simulink model "interface_model"  (R2017b)
settings: Solver=FixedStepDiscrete  StartTime=0.0  StopTime=inf  RelTol=1e-3
undefined symbols (not defined in the file or in its folder): ip
libraries: zynqradiolib x2
settings Model: Creator=tcollins  LastModifiedBy=tcollins

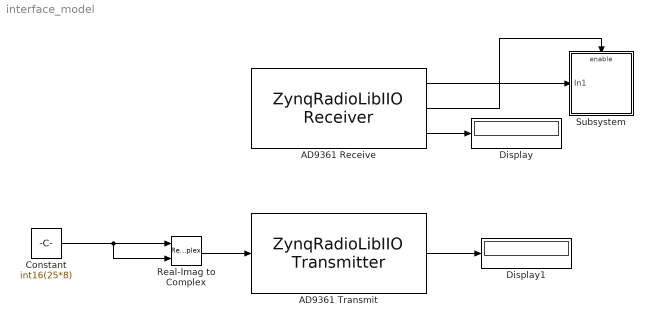
== system interface_model ==
  AD9361 Receive : zynqradiolib/ZynqRadioLibIIO Receiver  SourceLibraryInfo="This block requires <a href=\"http://www.mathworks.com/hardware-support/rtl-sdr.html\">Communications System Toolbox Support Package for RTL-SDR Radio</a>"  IPAddress=192.168.3.2  uri=ip:10.0.0.200  CenterFrequencySource=Dialog  CenterFrequency=2.4e9  GainSource=AGC Slow Attack  Gain=10  ChannelMapping=1  BasebandSampleRate=2e6  OutputDataType=int16  SamplesPerFrame=20000  OverflowOutputPort=on  ShowAdvancedProperties=off  Timeout=30  EnableQuadratureTracking=on  EnableRFDCTracking=on  EnableBasebandDCTracking=on  UseCustomFilter=off  filtPathRates=[ 737280000, 11520000, 3840000, 1920000, 960000, 240000 ]  filtCoefficients=round( fir1( 127, 0.75 )*2^15*10^1.2 )  filtCoefficientSize=128  filtDecimInterpFactor=4  filtGain=-12  filtRFBandwidth=18e6  filterConfigStruct=struct()  ENSMPinControlMode=None  BISTLoopbackMode=Disabled
  AD9361 Transmit : zynqradiolib/ZynqRadioLibIIO Transmitter  SourceLibraryInfo="This block requires <a href=\"http://www.mathworks.com/hardware-support/rtl-sdr.html\">Communications System Toolbox Support Package for RTL-SDR Radio</a>"  IPAddress=192.168.3.2  uri=ip:10.0.0.200  CenterFrequencySource=Dialog  CenterFrequency=2.4e9+0  GainSource=Dialog  Gain=-10  ChannelMapping=1  BasebandSampleRate=2e6  UnderflowOutputPort=on  ShowAdvancedProperties=off  Timeout=30  DataSourceSelect=Input Port  DDSTone1Freq=5e3  DDSTone2Freq=10e3  DDSTone1Scale=0.5  DDSTone2Scale=0.25  UseCustomFilter=off  filtPathRates=[ 737280000, 11520000, 3840000, 1920000, 960000, 240000 ]  filtCoefficients=round( fir1( 127, 0.75 )*2^15*10^1.2 )  filtCoefficientSize=128  filtDecimInterpFactor=4  filtGain=-12  filtRFBandwidth=18e6  filterConfigStruct=struct()  ENSMPinControlMode=None  BISTLoopbackMode=Disabled
  Constant : Constant  Value=int16(25*8)
  Display : Display
  Display1 : Display
  Real-Imag to Complex : RealImagToComplex
  Subsystem : Subsystem
  wires:
  Real-Imag to Complex/1 -> AD9361 Transmit/1
  Constant/1 -> Real-Imag to Complex/2, Real-Imag to Complex/1
  AD9361 Receive/1 -> Subsystem/1(In1)
  AD9361 Receive/2 -> Subsystem/Enable
  AD9361 Receive/3 -> Display/1
  AD9361 Transmit/1 -> Display1/1

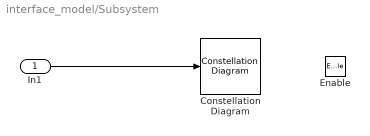
== system interface_model/Subsystem ==
  In1 : Inport
  Enable : EnablePort
  Constellation Diagram : ConstellationDiagram
  wires:
  In1/1 -> Constellation Diagram/1
